simulink model "udo10th"  (R2024b)
settings: Solver=FixedStepAuto  StartTime=0.0  StopTime=10.0  FixedStep=0.001  RelTol=1e-3
settings Model: Creator=user  LastModifiedBy=user

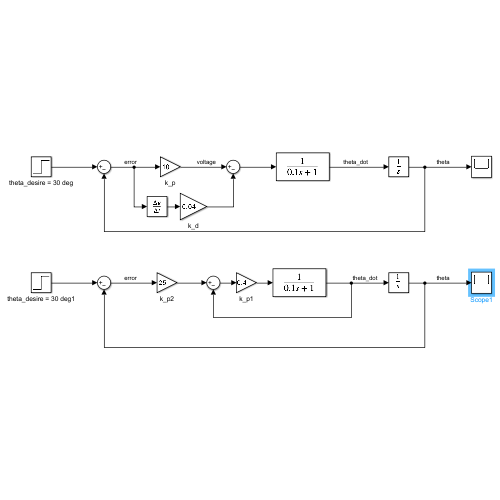
[thumbnail: Simulink's stored preview of the top-level diagram]
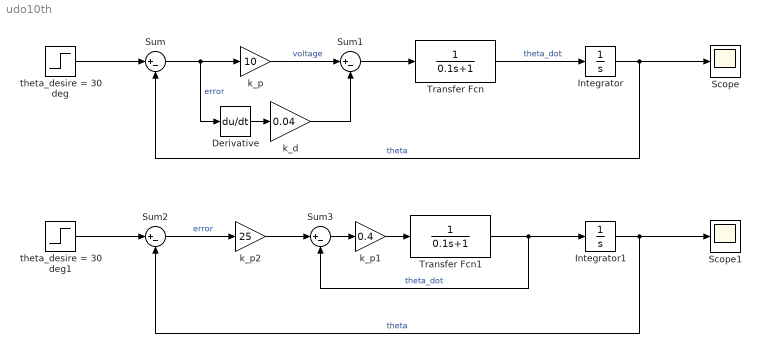
== system udo10th ==
  Derivative : Derivative
  Integrator : Integrator
  Integrator1 : Integrator
  Scope : Scope
  Scope1 : Scope
  Sum{,1..3} (4 alike) : Sum  Inputs=|+-
  Transfer Fcn : TransferFcn  Denominator=[0.1 1]
  Transfer Fcn1 : TransferFcn  Denominator=[0.1 1]
  k_d : Gain  Gain=0.04
  k_p : Gain  Gain=10
  k_p1 : Gain  Gain=0.4
  k_p2 : Gain  Gain=25
  theta_desire = 30 deg : Step  Time=0  After=30  SampleTime=0
  theta_desire = 30 deg1 : Step  Time=0  After=30  SampleTime=0
  wires:
  theta_desire = 30 deg/1 -> Sum/1
  Sum/1 -> Derivative/1, k_p/1  "error"
  k_p/1 -> Sum1/1  "voltage"
  Transfer Fcn/1 -> Integrator/1  "theta_dot"
  Integrator/1 -> Scope/1, Sum/2  "theta"
  Derivative/1 -> k_d/1
  k_d/1 -> Sum1/2
  Sum1/1 -> Transfer Fcn/1
  k_p2/1 -> Sum3/1
  Integrator1/1 -> Scope1/1, Sum2/2  "theta"
  theta_desire = 30 deg1/1 -> Sum2/1
  Sum2/1 -> k_p2/1  "error"
  Transfer Fcn1/1 -> Sum3/2, Integrator1/1  "theta_dot"
  Sum3/1 -> k_p1/1
  k_p1/1 -> Transfer Fcn1/1
